simulink model "PC_processing"  (R2020a)
settings: Solver=FixedStepDiscrete  StartTime=0.0  StopTime=P.t_end  FixedStep=P.dt  RelTol=1e-3
settings Model: Creator=divad  LastModifiedBy=divad
settings DataIOCC: SaveFormat=Structure  SaveOutput=off  SignalLogging=off  DSMLogging=off  SaveTime=off

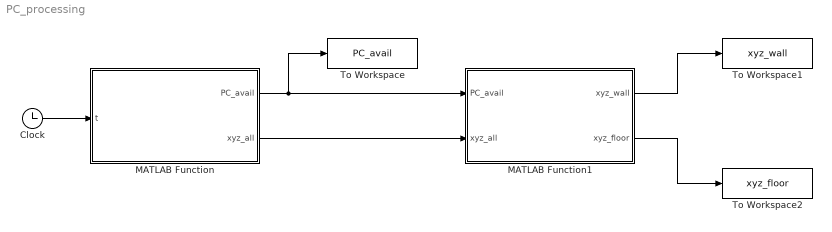
== system PC_processing ==
  Clock : Clock
  MATLAB Function : MATLAB Function  TreatAsAtomicUnit=on
  MATLAB Function1 : MATLAB Function  TreatAsAtomicUnit=on
  To Workspace : ToWorkspace  VariableName=PC_avail  SampleTime=-1
  To Workspace1 : ToWorkspace  VariableName=xyz_wall  SampleTime=-1
  To Workspace2 : ToWorkspace  VariableName=xyz_floor  SampleTime=-1
  wires:
  Clock/1 -> MATLAB Function/1(t)
  MATLAB Function/1(PC_avail) -> To Workspace/1, MATLAB Function1/1(PC_avail)
  MATLAB Function/2(xyz_all) -> MATLAB Function1/2(xyz_all)
  MATLAB Function1/1(xyz_wall) -> To Workspace1/1
  MATLAB Function1/2(xyz_floor) -> To Workspace2/1

== matlab function PC_processing/MATLAB Function ==
  data: t input; PC_avail output; P parameter; xyz_all output
function [PC_avail, xyz_all] = provide_point_cloud(t, P)

% Initialize Indexing Variable
persistent k 
if (isempty(k))
    k = 1;
end

% Provide Depth Data
if (mod(t,1) == 0)
    PC_avail = 1;
    xyz_all = P.xyz(:,:,k);
    k = k + 1;
else
    PC_avail = 0;
    xyz_all = zeros(3, 3072);
end

== matlab function PC_processing/MATLAB Function1 ==
  data: PC_avail input; xyz_wall output; xyz_all input; xyz_floor output
function [xyz_wall, xyz_floor] = split_wall_and_floor(PC_avail, xyz_all)

%% When a Point Cloud (PC) is available
if (PC_avail == 1)
    
    % Designate Wall/Floor Threshold
    wall_floor_threshold = 0; % meters
    floor_threshold = 1.5;    % meters
    
    % Pre-Allocate Memory
    xyz_wall = zeros(3, 3072);
    xyz_floor = zeros(3, 3072);
    
    % Separate Wall & Floor Points
    for k = 1 : length(xyz_all)
        
        % if xyz point is already zero
        if (norm(xyz_all(:,k)) < 0.05)
            xyz_wall(:,k) = [0; 0; 0];
            xyz_floor(:,k) = [0; 0; 0];
        elseif (xyz_all(3,k) >= wall_floor_threshold)
            xyz_wall(:,k) = xyz_all(:,k);
            xyz_floor(:,k) = [0; 0; 0];
        elseif ((xyz_all(3,k) < wall_floor_threshold) && (xyz_all(1,k) < floor_threshold))
            xyz_wall(:,k) = [0; 0; 0];
            xyz_floor(:,k) = xyz_all(:,k);
        end
        
    end
    
else
    
    % Send all zeros matrix
    xyz_wall = zeros(3, 3072);
    xyz_floor = zeros(3, 3072);
    
end
